simulink model "lqr_model"  (R2024a)
settings: Solver=FixedStepAuto  StartTime=0.0  StopTime=8  FixedStep=0.0001  MinStep=1e-8  RelTol=1e-8  AbsTol=1e-8
values from neighbouring files (symbols this model uses):
  A = A1 + A2 + A3    [graphs.m]    (also in lqr.m = [0 1; 5 -4]; lqr1.m = [0 1; 5 -4]; lqr2.m = [0 1; 5 -4]; lqr3.m = [0 1; 5 -4])
  b = [1; 1]    [lqr.m]    (also in lqr1.m; lqr2.m; lqr3.m)
  K1 = [2 0.525]    [lqr1.m]
  K2 = [1.7 0.35]    [lqr2.m]
  x0 = [0; 0]    [graphs.m]    (also in lqr.m = [1; 0]; lqr1.m = [1; 0]; lqr2.m = [1; 0]; lqr3.m = [1; 0])
undefined symbols (not defined in the file or in its folder): K, K3
settings Model: Creator=ventus  LastModifiedBy=ventus

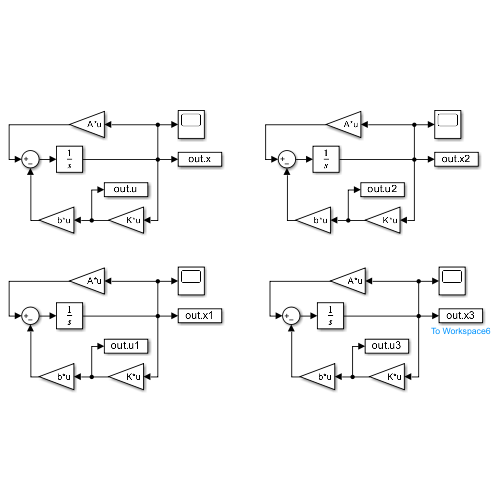
[thumbnail: Simulink's stored preview of the top-level diagram]
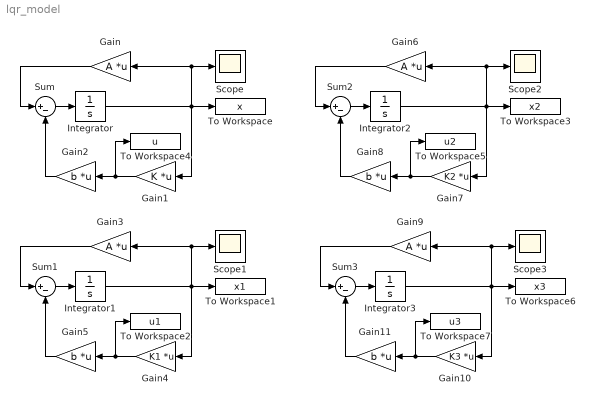
== system lqr_model ==
  Gain{,3,6,9} (4 alike) : Gain  Gain=A  Multiplication=Matrix(K*u)
  Gain1 : Gain  Gain=K  Multiplication=Matrix(K*u)
  Gain10 : Gain  Gain=K3  Multiplication=Matrix(K*u)
  Gain{2,5,8,11} (4 alike) : Gain  Gain=b  Multiplication=Matrix(K*u)
  Gain4 : Gain  Gain=K1  Multiplication=Matrix(K*u)
  Gain7 : Gain  Gain=K2  Multiplication=Matrix(K*u)
  Integrator{,1..3} (4 alike) : Integrator  InitialCondition=x0
  Scope{,1..3} (4 alike) : Scope
  Sum{,1..3} (4 alike) : Sum  Inputs=|+-
  To Workspace : ToWorkspace  VariableName=x  SaveFormat=Timeseries  SampleTime=-1
  To Workspace1 : ToWorkspace  VariableName=x1  SaveFormat=Timeseries  SampleTime=-1
  To Workspace2 : ToWorkspace  VariableName=u1  SaveFormat=Timeseries  SampleTime=-1
  To Workspace3 : ToWorkspace  VariableName=x2  SaveFormat=Timeseries  SampleTime=-1
  To Workspace4 : ToWorkspace  VariableName=u  SaveFormat=Timeseries  SampleTime=-1
  To Workspace5 : ToWorkspace  VariableName=u2  SaveFormat=Timeseries  SampleTime=-1
  To Workspace6 : ToWorkspace  VariableName=x3  SaveFormat=Timeseries  SampleTime=-1
  To Workspace7 : ToWorkspace  VariableName=u3  SaveFormat=Timeseries  SampleTime=-1
  wires:
  Integrator/1 -> Gain/1, Scope/1, To Workspace/1, Gain1/1
  Sum/1 -> Integrator/1
  Gain/1 -> Sum/1
  Gain1/1 -> Gain2/1, To Workspace4/1
  Gain2/1 -> Sum/2
  Gain4/1 -> Gain5/1, To Workspace2/1
  Integrator1/1 -> Scope1/1, Gain3/1, To Workspace1/1, Gain4/1
  Gain5/1 -> Sum1/2
  Gain3/1 -> Sum1/1
  Sum1/1 -> Integrator1/1
  Gain6/1 -> Sum2/1
  Sum2/1 -> Integrator2/1
  Gain8/1 -> Sum2/2
  Integrator2/1 -> Scope2/1, Gain6/1, To Workspace3/1, Gain7/1
  Gain7/1 -> Gain8/1, To Workspace5/1
  Gain9/1 -> Sum3/1
  Sum3/1 -> Integrator3/1
  Gain11/1 -> Sum3/2
  Integrator3/1 -> Scope3/1, Gain9/1, To Workspace6/1, Gain10/1
  Gain10/1 -> Gain11/1, To Workspace7/1
